simulink model "compartment"  (R2020b)
settings: Solver=VariableStepAuto  StartTime=0.0  StopTime=10.0  RelTol=1e-3
values from neighbouring files (symbols this model uses):
  a0 = 0.2    [compartment_script.m]
  a1 = 0.1    [compartment_script.m]
  a2 = 0.3    [compartment_script.m]
  b = 1    [compartment_script.m]
settings Model: Creator=kjartan  LastModifiedBy=kjartan

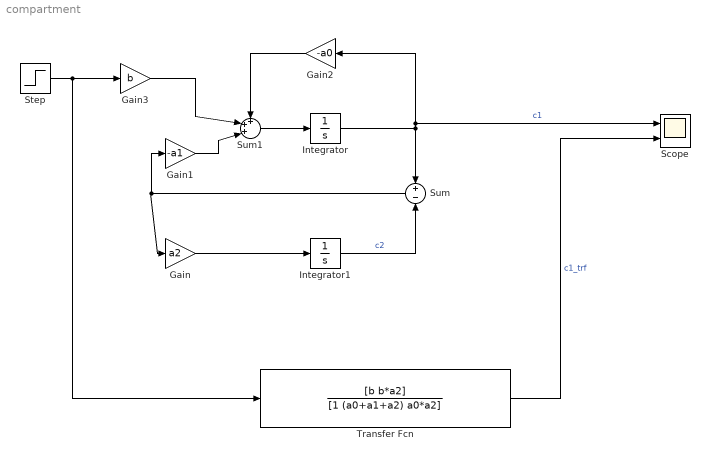
== system compartment ==
  Gain : Gain  Gain=a2
  Gain1 : Gain  Gain=-a1
  Gain2 : Gain  Gain=-a0
  Gain3 : Gain  Gain=b
  Integrator : Integrator
  Integrator1 : Integrator
  Scope : Scope  NumInputPorts=2
  Step : Step  SampleTime=0
  Sum : Sum  Inputs=+|-
  Sum1 : Sum  Inputs=+++|
  Transfer Fcn : TransferFcn  Numerator=[b b*a2]  Denominator=[1 (a0+a1+a2) a0*a2]
  wires:
  Integrator1/1 -> Sum/2  "c2"
  Integrator/1 -> Sum/1, Gain2/1, Scope/1  "c1"
  Gain/1 -> Integrator1/1
  Gain1/1 -> Sum1/3
  Sum/1 -> Gain1/1, Gain/1
  Sum1/1 -> Integrator/1
  Gain2/1 -> Sum1/1
  Step/1 -> Transfer Fcn/1, Gain3/1
  Gain3/1 -> Sum1/2
  Transfer Fcn/1 -> Scope/2  "c1_trf"
